simulink model "updated_target_driver_2026_withVariants_MPC"  (R2024b)
settings: Solver=FixedStepDiscrete  StartTime=0.0  StopTime=running_time  FixedStep=dt_s  RelTol=1e-3
values from neighbouring files (symbols this model uses):
  A = gamma_2*gamma_3*Thrust_desired    [force2voltage.m]
  a2_lb = -0.25    [target_driver_setup_2022_Ctrl_V_2_4.m]    (also in target_driver_setup_2022_Ctrl_V_2_4_geometric.m; target_driver_setup_mpc_12msdelay.m; target_driver_setup_mpc_andWLQP.m)
  a2_openloop = -0    (= 0)    [target_driver_setup_2022_Ctrl_V_2_4.m]    (also in target_driver_setup_2022_Ctrl_V_2_4_geometric.m; target_driver_setup_mpc_12msdelay.m; target_driver_setup_mpc_andWLQP.m)
  a2_ub = 0.25    [target_driver_setup_2022_Ctrl_V_2_4.m]    (also in target_driver_setup_2022_Ctrl_V_2_4_geometric.m; target_driver_setup_mpc_12msdelay.m; target_driver_setup_mpc_andWLQP.m)
  adaptive_flag = 0    [target_driver_setup_2022_Ctrl_V_2_4.m]    (also in target_driver_setup_2022_Ctrl_V_2_4_geometric.m; target_driver_setup_mpc_12msdelay.m = 1; target_driver_setup_mpc_andWLQP.m = 1)
  adaptive_gain = [gamma_adaptive, adaptive_roll_limit, adaptive_pitch_limit, adaptive_yaw_limit, c_2_adaptive, gamma_lateral_adaptive, adaptive_x_limit, adaptive_y_limit, adaptive_z_limit, c_1_adaptive]    [target_driver_setup_2022_Ctrl_V_2_4.m]    (also in target_driver_setup_2022_Ctrl_V_2_4_geometric.m; target_driver_setup_mpc_12msdelay.m; target_driver_setup_mpc_andWLQP.m)
  adaptive_lateral_flag = 0    [target_driver_setup_2022_Ctrl_V_2_4.m]    (also in target_driver_setup_2022_Ctrl_V_2_4_geometric.m; target_driver_setup_mpc_12msdelay.m = 1; target_driver_setup_mpc_andWLQP.m = 1)
  adaptive_pitch_init = 0    [target_driver_setup_2022_Ctrl_V_2_4.m]    (also in target_driver_setup_2022_Ctrl_V_2_4_geometric.m; target_driver_setup_mpc_12msdelay.m; target_driver_setup_mpc_andWLQP.m)
  adaptive_pitch_limit = 0.1/(scale^2)    (= 1e-07)    [target_driver_setup_2022_Ctrl_V_2_4.m]    (also in target_driver_setup_2022_Ctrl_V_2_4_geometric.m = 3e-07; target_driver_setup_mpc_12msdelay.m; target_driver_setup_mpc_andWLQP.m)
  adaptive_pitch_limit_low = -adaptive_pitch_limit    (= -1e-07)    [target_driver_setup_2022_Ctrl_V_2_4.m]    (also in target_driver_setup_2022_Ctrl_V_2_4_geometric.m = -3e-07; target_driver_setup_mpc_12msdelay.m; target_driver_setup_mpc_andWLQP.m)
  adaptive_roll_init = 0    [target_driver_setup_2022_Ctrl_V_2_4.m]    (also in target_driver_setup_2022_Ctrl_V_2_4_geometric.m; target_driver_setup_mpc_12msdelay.m; target_driver_setup_mpc_andWLQP.m)
  adaptive_roll_limit = 0.3/(scale^2)    (= 3e-07)    [target_driver_setup_2022_Ctrl_V_2_4.m]    (also in target_driver_setup_2022_Ctrl_V_2_4_geometric.m; target_driver_setup_mpc_12msdelay.m; target_driver_setup_mpc_andWLQP.m)
  adaptive_roll_limit_low = -adaptive_roll_limit    (= -3e-07)    [target_driver_setup_2022_Ctrl_V_2_4.m]    (also in target_driver_setup_2022_Ctrl_V_2_4_geometric.m; target_driver_setup_mpc_12msdelay.m; target_driver_setup_mpc_andWLQP.m)
  adaptive_x_init = 0    [target_driver_setup_2022_Ctrl_V_2_4.m]    (also in target_driver_setup_2022_Ctrl_V_2_4_geometric.m; target_driver_setup_mpc_12msdelay.m; target_driver_setup_mpc_andWLQP.m)
  adaptive_x_limit = 0.15/(scale)    (= 0.00015)    [target_driver_setup_2022_Ctrl_V_2_4.m]    (also in target_driver_setup_2022_Ctrl_V_2_4_geometric.m = 7.5e-05; target_driver_setup_mpc_12msdelay.m; target_driver_setup_mpc_andWLQP.m)
  adaptive_x_limit_low = -adaptive_x_limit    (= -0.00015)    [target_driver_setup_2022_Ctrl_V_2_4.m]    (also in target_driver_setup_2022_Ctrl_V_2_4_geometric.m = -7.5e-05; target_driver_setup_mpc_12msdelay.m; target_driver_setup_mpc_andWLQP.m)
  adaptive_y_init = 0    [target_driver_setup_2022_Ctrl_V_2_4.m]    (also in target_driver_setup_2022_Ctrl_V_2_4_geometric.m; target_driver_setup_mpc_12msdelay.m; target_driver_setup_mpc_andWLQP.m)
  adaptive_y_limit = 0.15/(scale)    (= 0.00015)    [target_driver_setup_2022_Ctrl_V_2_4.m]    (also in target_driver_setup_2022_Ctrl_V_2_4_geometric.m = 7.5e-05; target_driver_setup_mpc_12msdelay.m; target_driver_setup_mpc_andWLQP.m)
  adaptive_y_limit_low = -adaptive_y_limit    (= -0.00015)    [target_driver_setup_2022_Ctrl_V_2_4.m]    (also in target_driver_setup_2022_Ctrl_V_2_4_geometric.m = -7.5e-05; target_driver_setup_mpc_12msdelay.m; target_driver_setup_mpc_andWLQP.m)
  adaptive_yaw_init = 0    [target_driver_setup_2022_Ctrl_V_2_4.m]    (also in target_driver_setup_2022_Ctrl_V_2_4_geometric.m; target_driver_setup_mpc_12msdelay.m; target_driver_setup_mpc_andWLQP.m)
  adaptive_yaw_limit = 0.035/(scale^2)    (= 3.5e-08)    [target_driver_setup_2022_Ctrl_V_2_4.m]    (also in target_driver_setup_2022_Ctrl_V_2_4_geometric.m; target_driver_setup_mpc_12msdelay.m; target_driver_setup_mpc_andWLQP.m)
  adaptive_yaw_limit_low = -adaptive_yaw_limit    (= -3.5e-08)    [target_driver_setup_2022_Ctrl_V_2_4.m]    (also in target_driver_setup_2022_Ctrl_V_2_4_geometric.m; target_driver_setup_mpc_12msdelay.m; target_driver_setup_mpc_andWLQP.m)
  adaptive_z_init = 0/scale    (= 0)    [target_driver_setup_2022_Ctrl_V_2_4.m]    (also in target_driver_setup_2022_Ctrl_V_2_4_geometric.m; target_driver_setup_mpc_12msdelay.m; target_driver_setup_mpc_andWLQP.m)
  adaptive_z_limit = 0.20/(scale)    (= 0.0002)    [target_driver_setup_2022_Ctrl_V_2_4.m]    (also in target_driver_setup_2022_Ctrl_V_2_4_geometric.m = 0.0008; target_driver_setup_mpc_12msdelay.m = 0.0008; target_driver_setup_mpc_andWLQP.m = 0.0008)
  adaptive_z_limit_low = -adaptive_z_limit/1    (= -0.0002)    [target_driver_setup_2022_Ctrl_V_2_4.m]    (also in target_driver_setup_2022_Ctrl_V_2_4_geometric.m = -0.0008; target_driver_setup_mpc_12msdelay.m = -0.0008; target_driver_setup_mpc_andWLQP.m = -0.0008)
  att_s = 500    [target_driver_setup_2022_Ctrl_V_2_4.m]    (also in target_driver_setup_2022_Ctrl_V_2_4_geometric.m; target_driver_setup_mpc_12msdelay.m; target_driver_setup_mpc_andWLQP.m)
  b_1_d_desired = [1,0,0]    [target_driver_setup_2022_Ctrl_V_2_4.m]    (also in target_driver_setup_2022_Ctrl_V_2_4_geometric.m; target_driver_setup_mpc_12msdelay.m; target_driver_setup_mpc_andWLQP.m)
  closedloop_flag = 1    [target_driver_setup_2022_Ctrl_V_2_4.m]    (also in target_driver_setup_2022_Ctrl_V_2_4_geometric.m = 0; target_driver_setup_mpc_12msdelay.m = 0; target_driver_setup_mpc_andWLQP.m = 0)
  control_gain = [k_x,k_v, k_R, k_Omega, k_z, k_vz, k_Rx]    [target_driver_setup_2022_Ctrl_V_2_4.m]    (also in target_driver_setup_2022_Ctrl_V_2_4_geometric.m = [k_x,k_v,k_R,k_Omega_pitch,k_Omega_roll,k_z,k_vz,k_Rx]; target_driver_setup_mpc_12msdelay.m = [k_x, k_v, k_R, k_Omega, k_z, k_vz, k_Rx,                  k; target_driver_setup_mpc_andWLQP.m = [k_x, k_v, k_R, k_Omega, k_z, k_vz, k_Rx,                  k)
  delay = delay-vicon_sample_cycle/2    [target_driver_setup_2022_Ctrl_V_2_4.m]    (also in target_driver_setup_2022_Ctrl_V_2_4_geometric.m; target_driver_setup_mpc_12msdelay.m; target_driver_setup_mpc_andWLQP.m)
  drv_amp = abs((vleft_p2p-vright_p2p))/2+min(vleft_p2p,vright_p2p)    [Wing_traj_to_Voltage.m]    (also in force2voltage.m; target_driver_setup_2022_Ctrl_V_2_4.m = 300; target_driver_setup_2022_Ctrl_V_2_4_geometric.m = 133; target_driver_setup_mpc_12msdelay.m = 150)
  drv_bias = max_drv_bias    (= 300)    [target_driver_setup_2022_Ctrl_V_2_4.m]    (also in target_driver_setup_2022_Ctrl_V_2_4_geometric.m = 200; target_driver_setup_mpc_12msdelay.m = 200; target_driver_setup_mpc_andWLQP.m = 200)
  drv_pitch_left = vleft_pitch    [Wing_traj_to_Voltage.m]    (also in force2voltage.m = 0; target_driver_setup_2022_Ctrl_V_2_4.m = 0; target_driver_setup_2022_Ctrl_V_2_4_geometric.m = 0; target_driver_setup_mpc_12msdelay.m = 9.05)
  drv_pitch_right = vright_pitch    [Wing_traj_to_Voltage.m]    (also in force2voltage.m = 0; target_driver_setup_2022_Ctrl_V_2_4.m = 0; target_driver_setup_2022_Ctrl_V_2_4_geometric.m = 0; target_driver_setup_mpc_12msdelay.m = 9.05)
  drv_roll = (vleft_p2p-vright_p2p)/4    [Wing_traj_to_Voltage.m]    (also in force2voltage.m; target_driver_setup_2022_Ctrl_V_2_4.m = 0; target_driver_setup_2022_Ctrl_V_2_4_geometric.m = -0.001; target_driver_setup_mpc_12msdelay.m = -0.001)
  dt_s = 1e-3    (= 0.001)    [target_driver_setup_2022_Ctrl_V_2_4.m]    (also in target_driver_setup_2022_Ctrl_V_2_4_geometric.m = 0.0002; target_driver_setup_mpc_12msdelay.m = 0.0002; target_driver_setup_mpc_andWLQP.m = 0.0002)
  f_fin = f    (= 180)    [target_driver_setup_2022_Ctrl_V_2_4.m]    (also in target_driver_setup_2022_Ctrl_V_2_4_geometric.m = 155; target_driver_setup_mpc_12msdelay.m = 155; target_driver_setup_mpc_andWLQP.m = 155)
  f_int = f    (= 180)    [target_driver_setup_2022_Ctrl_V_2_4.m]    (also in target_driver_setup_2022_Ctrl_V_2_4_geometric.m = 155; target_driver_setup_mpc_12msdelay.m = 155; target_driver_setup_mpc_andWLQP.m = 155)
  g = 9.8    [target_driver_setup_2022_Ctrl_V_2_4.m]    (also in target_driver_setup_2022_Ctrl_V_2_4_geometric.m; target_driver_setup_mpc_12msdelay.m; target_driver_setup_mpc_andWLQP.m = 9.81; test_full_attitude_mpc.m = 9.81)
  I_moment_vec = [Ixx, Iyy, Izz]    [target_driver_setup_2022_Ctrl_V_2_4.m]    (also in target_driver_setup_2022_Ctrl_V_2_4_geometric.m; target_driver_setup_mpc_12msdelay.m; target_driver_setup_mpc_andWLQP.m)
  k_tau_vec = [k_tau_roll;k_tau_pitch]    [target_driver_setup_2022_Ctrl_V_2_4_geometric.m]    (also in target_driver_setup_mpc_12msdelay.m; target_driver_setup_mpc_andWLQP.m)
  landing_flag = 0    [target_driver_setup_2022_Ctrl_V_2_4.m]    (also in target_driver_setup_2022_Ctrl_V_2_4_geometric.m; target_driver_setup_mpc_12msdelay.m; target_driver_setup_mpc_andWLQP.m)
  landing_parameter = [start_delay+T,transition_rate, rising_time, falling_time, landing_rising_time, landing_z_decrease, landing_y_decrease, landing_x_decrease]    [target_driver_setup_2022_Ctrl_V_2_4.m]    (also in target_driver_setup_2022_Ctrl_V_2_4_geometric.m; target_driver_setup_mpc_12msdelay.m; target_driver_setup_mpc_andWLQP.m)
  low_bound = -8    [target_driver_setup_2022_Ctrl_V_2_4.m]    (also in target_driver_setup_2022_Ctrl_V_2_4_geometric.m = -5; target_driver_setup_mpc_12msdelay.m = -10; target_driver_setup_mpc_andWLQP.m = -10)
  low_bound_eR = -0.8    [target_driver_setup_2022_Ctrl_V_2_4.m]    (also in target_driver_setup_2022_Ctrl_V_2_4_geometric.m = -1.2; target_driver_setup_mpc_12msdelay.m = -1.2; target_driver_setup_mpc_andWLQP.m = -1.2)
  low_bound_vx = -0.5    [target_driver_setup_2022_Ctrl_V_2_4.m]    (also in target_driver_setup_2022_Ctrl_V_2_4_geometric.m; target_driver_setup_mpc_12msdelay.m; target_driver_setup_mpc_andWLQP.m)
  low_bound_vy = -0.5    [target_driver_setup_2022_Ctrl_V_2_4.m]    (also in target_driver_setup_2022_Ctrl_V_2_4_geometric.m; target_driver_setup_mpc_12msdelay.m; target_driver_setup_mpc_andWLQP.m)
  low_bound_vz = -0.5    [target_driver_setup_2022_Ctrl_V_2_4.m]    (also in target_driver_setup_2022_Ctrl_V_2_4_geometric.m; target_driver_setup_mpc_12msdelay.m; target_driver_setup_mpc_andWLQP.m)
  low_bound_x = -0.06    [target_driver_setup_2022_Ctrl_V_2_4.m]    (also in target_driver_setup_2022_Ctrl_V_2_4_geometric.m = -0.1; target_driver_setup_mpc_12msdelay.m = -0.6; target_driver_setup_mpc_andWLQP.m = -0.6)
  low_bound_y = -0.06    [target_driver_setup_2022_Ctrl_V_2_4.m]    (also in target_driver_setup_2022_Ctrl_V_2_4_geometric.m; target_driver_setup_mpc_12msdelay.m = -0.6; target_driver_setup_mpc_andWLQP.m = -0.6)
  low_bound_z = -0.04    [target_driver_setup_2022_Ctrl_V_2_4.m]    (also in target_driver_setup_2022_Ctrl_V_2_4_geometric.m; target_driver_setup_mpc_12msdelay.m = -0.1; target_driver_setup_mpc_andWLQP.m = -0.1)
  m = t <= t_zoom    [plot_roll_torque_cmd_vs_actual.m]    (also in plot_roll_torque_cmd_vs_actual_flightlog.m = t >= t0 & t <= t1; target_driver_setup_2022_Ctrl_V_2_4.m = 0.000124; target_driver_setup_2022_Ctrl_V_2_4_geometric.m = 8.5655e-05; target_driver_setup_mpc_12msdelay.m = 8.5655e-05)
  params_vec = [params_opt.delta_1, params_opt.delta_2, params_opt.delta_3,      params_opt.gamma_1, params_opt.gamma_2_1, params_opt.gamma_3,      params_opt.eta, params_opt.nu, params_opt.mu]'    [force2voltage_tuningSandbox.m]    (also in target_driver_setup_2022_Ctrl_V_2_4.m = [params_opt.delta_1, params_opt.delta_2, params_opt.delta_3,; target_driver_setup_2022_Ctrl_V_2_4_geometric.m = [params_opt.delta_1, params_opt.delta_2, params_opt.delta_3,; target_driver_setup_mpc_12msdelay.m = [params_opt.delta_1, params_opt.delta_2, params_opt.delta_3,; target_driver_setup_mpc_andWLQP.m = [params_opt.delta_1, params_opt.delta_2, params_opt.delta_3,)
  phase = 0    [target_driver_setup_2022_Ctrl_V_2_4.m]    (also in target_driver_setup_2022_Ctrl_V_2_4_geometric.m; target_driver_setup_mpc_12msdelay.m; target_driver_setup_mpc_andWLQP.m)
  r_desired = [default_x, default_y,z_desired]    [target_driver_setup_2022_Ctrl_V_2_4.m]    (also in target_driver_setup_2022_Ctrl_V_2_4_geometric.m; target_driver_setup_mpc_12msdelay.m; target_driver_setup_mpc_andWLQP.m)
  roll_offset_angle = 0    [target_driver_setup_2022_Ctrl_V_2_4.m]    (also in target_driver_setup_2022_Ctrl_V_2_4_geometric.m; target_driver_setup_mpc_12msdelay.m; target_driver_setup_mpc_andWLQP.m)
  running_time = start_delay+total_T    (= 9)    [target_driver_setup_2022_Ctrl_V_2_4.m]    (also in target_driver_setup_2022_Ctrl_V_2_4_geometric.m = 10; target_driver_setup_mpc_12msdelay.m = 0.5; target_driver_setup_mpc_andWLQP.m = 10)
  running_time_control = start_delay_control+total_T+0.0    (= 7.1)    [target_driver_setup_2022_Ctrl_V_2_4.m]    (also in target_driver_setup_2022_Ctrl_V_2_4_geometric.m = 10; target_driver_setup_mpc_12msdelay.m = 0.5; target_driver_setup_mpc_andWLQP.m = 10)
  sampling_f = 10000    [target_driver_setup_2022_Ctrl_V_2_4.m]    (also in target_driver_setup_2022_Ctrl_V_2_4_geometric.m = 5000; target_driver_setup_mpc_12msdelay.m = 5000; target_driver_setup_mpc_andWLQP.m = 5000)
  start_delay = 2.0    (= 2)    [target_driver_setup_2022_Ctrl_V_2_4.m]    (also in target_driver_setup_2022_Ctrl_V_2_4_geometric.m = 0; target_driver_setup_mpc_12msdelay.m = 0; target_driver_setup_mpc_andWLQP.m = 0)
  start_delay_control = start_delay + ramp_delay    (= 0.1)    [target_driver_setup_2022_Ctrl_V_2_4.m]    (also in target_driver_setup_2022_Ctrl_V_2_4_geometric.m = 0; target_driver_setup_mpc_12msdelay.m = 0; target_driver_setup_mpc_andWLQP.m = 0)
  T = 1    [target_driver_setup_2022_Ctrl_V_2_4.m]    (also in target_driver_setup_2022_Ctrl_V_2_4_geometric.m = 10; target_driver_setup_mpc_12msdelay.m = 0.5; target_driver_setup_mpc_andWLQP.m = 10; test_full_attitude_mpc.m = T0 + nu(1))
  task_flag = 0    [target_driver_setup_2022_Ctrl_V_2_4.m]    (also in target_driver_setup_2022_Ctrl_V_2_4_geometric.m; target_driver_setup_mpc_12msdelay.m; target_driver_setup_mpc_andWLQP.m)
  task_parameter = [radius_ref, frequency_ref, radius_ratio, lissajous_ratio, lissajous_delta, lissajous_amplitude_ratio,z_radius_ratio]    [target_driver_setup_2022_Ctrl_V_2_4.m]    (also in target_driver_setup_2022_Ctrl_V_2_4_geometric.m; target_driver_setup_mpc_12msdelay.m; target_driver_setup_mpc_andWLQP.m)
  upp_bound = 8    [target_driver_setup_2022_Ctrl_V_2_4.m]    (also in target_driver_setup_2022_Ctrl_V_2_4_geometric.m = 5; target_driver_setup_mpc_12msdelay.m = 10; target_driver_setup_mpc_andWLQP.m = 10)
  upp_bound_eR = 0.8    [target_driver_setup_2022_Ctrl_V_2_4.m]    (also in target_driver_setup_2022_Ctrl_V_2_4_geometric.m = 1.2; target_driver_setup_mpc_12msdelay.m = 1.2; target_driver_setup_mpc_andWLQP.m = 1.2)
  upp_bound_vx = 0.5    [target_driver_setup_2022_Ctrl_V_2_4.m]    (also in target_driver_setup_2022_Ctrl_V_2_4_geometric.m; target_driver_setup_mpc_12msdelay.m; target_driver_setup_mpc_andWLQP.m)
  upp_bound_vy = 0.5    [target_driver_setup_2022_Ctrl_V_2_4.m]    (also in target_driver_setup_2022_Ctrl_V_2_4_geometric.m; target_driver_setup_mpc_12msdelay.m; target_driver_setup_mpc_andWLQP.m)
  upp_bound_vz = 0.5    [target_driver_setup_2022_Ctrl_V_2_4.m]    (also in target_driver_setup_2022_Ctrl_V_2_4_geometric.m; target_driver_setup_mpc_12msdelay.m; target_driver_setup_mpc_andWLQP.m)
  upp_bound_x = 0.06    [target_driver_setup_2022_Ctrl_V_2_4.m]    (also in target_driver_setup_2022_Ctrl_V_2_4_geometric.m = 0.1; target_driver_setup_mpc_12msdelay.m = 0.6; target_driver_setup_mpc_andWLQP.m = 0.6)
  upp_bound_y = 0.06    [target_driver_setup_2022_Ctrl_V_2_4.m]    (also in target_driver_setup_2022_Ctrl_V_2_4_geometric.m; target_driver_setup_mpc_12msdelay.m = 0.6; target_driver_setup_mpc_andWLQP.m = 0.6)
  upp_bound_z = 0.04    [target_driver_setup_2022_Ctrl_V_2_4.m]    (also in target_driver_setup_2022_Ctrl_V_2_4_geometric.m; target_driver_setup_mpc_12msdelay.m = 0.1; target_driver_setup_mpc_andWLQP.m = 0.1)
  weights_vec = [ws; wds; wpr_xy;wpr_z; wpf; wvr_xy; wvr_z ... (first row only)    [target_driver_setup_2022_Ctrl_V_2_4_geometric.m]    (also in target_driver_setup_mpc_12msdelay.m; target_driver_setup_mpc_andWLQP.m)
undefined symbols (not defined in the file or in its folder): Com1, DiscIntNeverNeededParam, dspblkCoreblockFVToolHelper, gcbh, left_mapping, left_mapping_F_to_Phi, lp_den, lp_num, none, right_mapping, right_mapping_F_to_Phi, vlp_den, vlp_num
libraries: simulink x20, xpcseriallib x2, cstblocks x1, xpcnilib x1, xpcutilitieslib x1
(part 6 of 7)

== matlab function updated_target_driver_2026_withVariants_MPC/Trajectory_generation ==
  data: task_flag input; r_desired_total output; t input; v_desired_total output; x_d_ddot_total output; b_1_d_total output; com_desired input; b_1_d_desired input; task_parameter input; landing_parameter input; landing_flag input; b_1_d_previous input
function [r_desired_total, v_desired_total, x_d_ddot_total, b_1_d_total] = fcn(task_flag, t, com_desired, b_1_d_desired, task_parameter, landing_parameter, landing_flag, b_1_d_previous)
    % com_desired = desired center of mass 
    % b_1_d
	% 
	if task_flag == 1
		radius_ref = task_parameter(1);
		frequency_ref = task_parameter(2);
		r_desired = com_desired + radius_ref*[cos(frequency_ref*t);-sin(frequency_ref*t);0];
		v_desired = radius_ref*frequency_ref*[-sin(frequency_ref*t);-cos(frequency_ref*t);0];
		x_d_ddot  = radius_ref*frequency_ref^2*[-cos(frequency_ref*t);sin(frequency_ref*t);0];

		if radius_ref<1e-6
			b_1_d     = b_1_d_desired;
		else
			% Looking into the center
	% 		b_1_d     = (com_desired - r_desired)/norm(com_desired - r_desired);

			% Looking to the tangent

			b_1_d = v_desired/norm(v_desired);

			% Looking th camera
	% 		 b_1_d = b_1_d_desired;
		end

	elseif task_flag == 2 % Elipse
		radius_ref = task_parameter(1);
		frequency_ref = task_parameter(2);
		radius_ratio = task_parameter(3);

		r_desired = com_desired + radius_ref*[radius_ratio*cos(frequency_ref*t);-sin(frequency_ref*t);0];
		v_desired = radius_ref*frequency_ref*[-radius_ratio*sin(frequency_ref*t);-cos(frequency_ref*t);0];
		x_d_ddot  = radius_ref*frequency_ref^2*[-radius_ratio*cos(frequency_ref*t);-(-sin(frequency_ref*t));0];

		if radius_ref<1e-6
			b_1_d     = b_1_d_desired;
		else
			% Looking into the center
	% 		b_1_d     = (com_desired - r_desired)/norm(com_desired - r_desired);

			% Looking to the tangent

			b_1_d = v_desired/norm(v_desired);
		end
	elseif task_flag==3 % Vertical up and down with the landing
		radius_ref = task_parameter(1);
		frequency_ref = task_parameter(2);
		landing_time = landing_parameter(1);

		r_desired = com_desired + radius_ref*[0;0;sin(frequency_ref*(t-landing_time)-pi/2)];
		v_desired = radius_ref*frequency_ref*[0;0;cos(frequency_ref*(t-landing_time)-pi/2)];
		x_d_ddot  = radius_ref*frequency_ref^2*[0;0;-sin(frequency_ref*(t-landing_time)-pi/2)];

		if radius_ref<1e-6
			b_1_d     = b_1_d_desired;
		else
			% Looking into the center
	% 		b_1_d     = (com_desired - r_desired)/norm(com_desired - r_desired);

			% Looking to the tangent

	% 		b_1_d = v_desired/norm(v_desired);
			% Looking th camera
			 b_1_d = b_1_d_desired;
		end
	elseif task_flag==4 % circle in y-z landing
		radius_ref = task_parameter(1);
		frequency_ref = task_parameter(2);
		landing_time = landing_parameter(1);

		r_desired = com_desired + radius_ref*[0;cos(frequency_ref*(t-landing_time)-pi/2);sin(frequency_ref*(t-landing_time)-pi/2)];
		v_desired = radius_ref*frequency_ref*[0;-sin(frequency_ref*(t-landing_time)-pi/2);cos(frequency_ref*(t-landing_time)-pi/2)];
		x_d_ddot  = radius_ref*frequency_ref^2*[0;-cos(frequency_ref*(t-landing_time)-pi/2);-sin(frequency_ref*(t-landing_time)-pi/2)];

		if radius_ref<1e-6
			b_1_d     = b_1_d_desired;
		else
			% Looking into the center
	% 		b_1_d     = (com_desired - r_desired)/norm(com_desired - r_desired);

			% Looking to the tangent

	% 		b_1_d = v_desired/norm(v_desired);
			% Looking th camera
			 b_1_d = b_1_d_desired;
		end	
	elseif task_flag==5 % Lissajous curve in y-z landing
		radius_ref = task_parameter(1);
		frequency_ref = task_parameter(2);
		landing_time = landing_parameter(1);
		lissajous_ratio = task_parameter(4);
		lissajous_delta = task_parameter(5);
		lissajous_amplitude_ratio = task_parameter(6);

		r_desired = com_desired + radius_ref*[0;sin(frequency_ref*lissajous_ratio*(t-landing_time)+lissajous_delta)											;lissajous_amplitude_ratio*sin(frequency_ref*(t-landing_time))];
		v_desired = radius_ref*frequency_ref*[0;lissajous_ratio*cos(frequency_ref*lissajous_ratio*(t-landing_time)+lissajous_delta)			;lissajous_amplitude_ratio*cos(frequency_ref*(t-landing_time))];
		x_d_ddot  = radius_ref*frequency_ref^2*[0;-lissajous_ratio^2*sin(frequency_ref*lissajous_ratio*(t-landing_time)+lissajous_delta)	;-lissajous_amplitude_ratio*sin(frequency_ref*(t-landing_time))];

		if radius_ref<1e-6
			b_1_d     = b_1_d_desired;
		else

			% Looking th camera
			 b_1_d = b_1_d_desired;
		end

	elseif task_flag==6 % Elipse
		radius_ref = task_parameter(1);
		frequency_ref = task_parameter(2);
		radius_ratio = task_parameter(3);
		z_radius_ratio = task_parameter(7);

		r_desired = com_desired + radius_ref*[radius_ratio*cos(frequency_ref*t);-sin(frequency_ref*t);-z_radius_ratio*sin(frequency_ref*t)];
		v_desired = radius_ref*frequency_ref*[-radius_ratio*sin(frequency_ref*t);-cos(frequency_ref*t);-z_radius_ratio*cos(frequency_ref*t)];
		x_d_ddot  = radius_ref*frequency_ref^2*[-radius_ratio*cos(frequency_ref*t);-(-sin(frequency_ref*t));-z_radius_ratio*(-sin(frequency_ref*t))];

		if radius_ref<1e-6
			b_1_d     = b_1_d_desired;
		else
			% Looking into the center
	% 		b_1_d     = (com_desired - r_desired)/norm(com_desired - r_desired);

			% Looking to the tangent

			b_1_d = v_desired/norm(v_desired);
		end	

	elseif task_flag==7 % Elipse
		radius_ref = task_parameter(1);
		heading_vector = [0;-1;0];

		r_desired = com_desired + radius_ref*heading_vector;
		v_desired = [0;0;0];
		x_d_ddot  = [0;0;0];

		if radius_ref<1e-6
			b_1_d     = b_1_d_desired;
		else
			% Looking into the center
	% 		b_1_d     = (com_desired - r_desired)/norm(com_desired - r_desired);

			% Looking to the tangent

	% 		b_1_d = v_desired/norm(v_desired);
			% Looking at the camera
			b_1_d     = b_1_d_desired;

		end		
	elseif task_flag==8
		landing_y_decrease = landing_parameter(7);
		landing_x_decrease = landing_parameter(8);

		r_desired = com_desired+[landing_x_decrease;landing_y_decrease;0];
		v_desired = [0;0;0];
		x_d_ddot  = [0;0;0];
		b_1_d     = b_1_d_desired;

	else
		r_desired = com_desired;
		v_desired = [0;0;0];
		x_d_ddot  = [0;0;0];
		b_1_d     = b_1_d_desired;
	end

	if landing_flag==1

		trans_rate=landing_parameter(2);
		rising_time =landing_parameter(3);
		falling_time =landing_parameter(4);
		landing_rising_time = landing_parameter(5);
		landing_z_decrease = landing_parameter(6);
		landing_y_decrease = landing_parameter(7);
		landing_x_decrease = landing_parameter(8);

	% Referenece trajectory band-pass

		if task_flag==8
			rising_func = (1+tanh(trans_rate*(t-rising_time)))/2;
			fallilng_func = 0;

		else
			rising_func = (1+tanh(trans_rate*(t-rising_time)))/2-1/2;
			fallilng_func = (1-tanh(trans_rate*(t-falling_time)))/2-1/2;

		end

		landing_rising_func = (1+tanh(trans_rate*(t-landing_rising_time)))/2;

		bandpass_func = rising_func+fallilng_func;
		neg_bandpass_func = -bandpass_func+1;

		der_bandpass_func = trans_rate*(1 -(tanh(trans_rate*(t-rising_time))).^2)/2 -trans_rate*(1-(tanh(trans_rate*(t-falling_time))).^2)/2;
		dder_bandpass_func = -2*trans_rate^2*(tanh(trans_rate*(t-rising_time))).*(1 -(tanh(trans_rate*(t-rising_time))).^2)/2 +2*trans_rate^2*(tanh(trans_rate*(t-falling_time))).*(1-(tanh(trans_rate*(t-falling_time))).^2)/2;

		der_landing_func = trans_rate*(1 -(tanh(trans_rate*(t-landing_rising_time))).^2)/2;
		dder_landing_func = -2*trans_rate^2*(tanh(trans_rate*(t-landing_rising_time))).*(1 -(tanh(trans_rate*(t-landing_rising_time))).^2)/2;

		landing_desired = com_desired+[landing_x_decrease;landing_y_decrease;landing_z_decrease];
	% 	landing_desired = com_desired+[0;0;landing_z_decrease];

		if task_flag==8 % Landing only z direction at r_desired point
			r_desired_total = com_desired + bandpass_func.*(r_desired-com_desired)+landing_rising_func.*(landing_desired-r_desired);
		else
			r_desired_total = com_desired + bandpass_func.*(r_desired-com_desired)+landing_rising_func.*(landing_desired-com_desired);	
		end

		v_desired_total = der_bandpass_func.*(r_desired-com_desired) + bandpass_func.*v_desired + der_landing_func.*(landing_desired-com_desired);
		x_d_ddot_total = dder_bandpass_func.*(r_desired-com_desired) + 2*der_bandpass_func.*v_desired+ bandpass_func.*x_d_ddot+ dder_landing_func.*(landing_desired-com_desired);

	% Heading trajectory band-pass
		trans_heading_rate = trans_rate*1/1;
		rising_heading_func = (1+tanh(trans_heading_rate*(t-(rising_time+1))))/2-1/2;
		fallilng_heading_func = (1-tanh(trans_heading_rate*(t-falling_time+1)))/2-1/2;
	% rising_heading_func = (1+tanh(trans_heading_rate*(t-(rising_time))))/2-1/2;
	% 	fallilng_heading_func = (1-tanh(trans_heading_rate*(t-falling_time)))/2-1/2;


		bandpass_heading_func = rising_heading_func+fallilng_heading_func;
		neg_bandpass_heading_func = -bandpass_heading_func+1;
		landing_rising_heading_func = (1+tanh(trans_heading_rate*(t-landing_rising_time)))/2;
	% 
	% 	if norm(v_desired_total)<1e-6
	% 		b_1_d     = b_1_d_desired;
	% 	else
	% 		b_1_d = v_desired_total/norm(v_desired_total);
	% 	end
	% 	
	% 	b_1_d_total = b_1_d_desired.*neg_bandpass_heading_func + b_1_d.*bandpass_heading_func;
	% 	
	% 	b_1_d_total = b_1_d_total/norm(b_1_d_total);
	% 	
	% 		% Convex combination of the heading vector
	% 	% Linear convex comb
	% 	b_1_d_total = b_1_d_desired.*neg_bandpass_func + b_1_d.*bandpass_func;


	% Slerp for smooth heading transition
	% STEP 1 : Hovering to Desired trajectory to Hovering

		if t<rising_time && bandpass_heading_func<1e-5%1e-6
			b_1_d_current = b_1_d_desired;
		else
			b_1_d_current = b_1_d_previous;
		end


		cos_Omega_slerp = b_1_d.'*b_1_d_current;
		Omega_slerp = acos(cos_Omega_slerp);

		if Omega_slerp<1e-8
			b_1_d_total = b_1_d_current.*neg_bandpass_heading_func + b_1_d.*bandpass_heading_func;
		else
			b_1_d_total = sin(neg_bandpass_heading_func*Omega_slerp)/sin(Omega_slerp)*b_1_d_current + sin(bandpass_heading_func*Omega_slerp)/sin(Omega_slerp)*b_1_d;
		end

	% STEP 2 : Hovering to Desired Heading for landing

		b_1_d_total = sin(1-landing_rising_heading_func)*b_1_d_total + sin(landing_rising_heading_func)*b_1_d_desired;

		b_1_d_total = b_1_d_total/norm(b_1_d_total);

	else
		r_desired_total = r_desired;
		v_desired_total = v_desired;
		x_d_ddot_total = x_d_ddot;
		b_1_d_total = b_1_d;

	end
end

== matlab function updated_target_driver_2026_withVariants_MPC/Force_to_Voltage1/Trajectory to Voltage Input  ==
  data: Phi_left_p2p_command input; drv_amp output; Phi_right_p2p_command input; Phi_pitch_command input; drv_roll output; drv_pitch_left output; left_mapping input; right_mapping input; drv_pitch_right output
function [drv_amp, drv_roll, drv_pitch_left, drv_pitch_right] = fcn(Phi_left_p2p_command,Phi_right_p2p_command,Phi_pitch_command,left_mapping,right_mapping)

% Mapping for Voltage peak to peak from desired Stroke peak to peak
p1_left = left_mapping(1); % V_left_p2p = p1_left*Phi_p2p + p2_left
p2_left = left_mapping(2);
p1_right = right_mapping(1); % V_right_p2p = p1_right*Phi_p2p + p2_right
p2_right = right_mapping(2);

% Mapping for Voltage offset to peak from desired Stroke peak to peak
p1_pitch_left = left_mapping(3); % vleft_pitch = p1_pitch_left*Phi_pitch_command + p2_pitch_left
p2_pitch_left = left_mapping(4);
p1_pitch_right = right_mapping(3); % vright_pitch = p1_pitch_right*Phi_pitch_command + p2_pitch_right
p2_pitch_right = right_mapping(4);

vleft_p2p = p1_left*Phi_left_p2p_command + p2_left;
vright_p2p = p1_right*Phi_right_p2p_command + p2_right;
vleft_pitch = p1_pitch_left*Phi_pitch_command + p2_pitch_left;
vright_pitch = p1_pitch_right*Phi_pitch_command + p2_pitch_right;



drv_amp = abs((vleft_p2p-vright_p2p))/2+min(vleft_p2p,vright_p2p); % p2p
drv_roll = (vleft_p2p-vright_p2p)/4; % Amplitude
drv_pitch_left = vleft_pitch;
drv_pitch_right = vright_pitch;

== matlab function updated_target_driver_2026_withVariants_MPC/Observer for averaged system1/Attitude Observer/Geometric Averaging Rotation Matix/Averaged quaternion ==
  data: R input; quat output
function quat = fcn(R)
Rot = zeros(3,3);
Rot = [R(1), R(2), R(3); R(4), R(5), R(6); R(7), R(8), R(9); ];
quat = rotm2quat(Rot)';

== matlab function updated_target_driver_2026_withVariants_MPC/Observer for averaged system1/Attitude Observer/Geometric Averaging Rotation Matix/Geometric Averaging Rotation M/Geometric Average  ==
  data: R_prev input; R_prev2 input; R_prev3 input; R_prev4 input; R_prev5 input; R_prev6 input; Rout output; R_cur input; update input; Rout_prev input
function Rout = fcn(R_prev,R_prev2,R_prev3,R_prev4,R_prev5,R_prev6,R_cur,update,Rout_prev)
%#codegen
% Average recent rotation matrices safely near small angles.
%
% Inputs are 9-vectors using row-major packing:
% R_vec = [R(1,1); R(1,2); R(1,3);
%          R(2,1); R(2,2); R(2,3);
%          R(3,1); R(3,2); R(3,3)]
%
% Output uses the same row-major packing.

Rout = zeros(9,1);

R_cur      = reshape(R_cur,9,1);
R_prev     = reshape(R_prev,9,1);
R_prev2    = reshape(R_prev2,9,1);
R_prev3    = reshape(R_prev3,9,1);
R_prev4    = reshape(R_prev4,9,1); %#ok<NASGU>
R_prev5    = reshape(R_prev5,9,1); %#ok<NASGU>
R_prev6    = reshape(R_prev6,9,1); %#ok<NASGU>
Rout_prev  = reshape(Rout_prev,9,1);

% Reconstruct row-major 9-vector into 3x3 matrix.
Rot_cur   = vec_to_rotm(R_cur);
Rot_prev  = vec_to_rotm(R_prev);
Rot_prev2 = vec_to_rotm(R_prev2);
Rot_prev3 = vec_to_rotm(R_prev3);

if update > 0
    Rout = Rout_prev;
else
    % 1-cycle / 4-sample average.
    %
    % IMPORTANT:
    % Do not do sign correction like w = -w here.
    % That is valid for quaternions, but not for rotation vectors.
    w_R0 = log_so3(Rot_cur);
    w_R1 = log_so3(Rot_prev);
    w_R2 = log_so3(Rot_prev2);
    w_R3 = log_so3(Rot_prev3);

    w_mean = (w_R0 + w_R1 + w_R2 + w_R3) / 4.0;

    mean_R = exp_so3(w_mean);

    % Optional but useful: project back to SO(3) to remove tiny numerical drift.
    mean_R = project_to_so3(mean_R);

    Rout = rotm_to_vec(mean_R);
end

end


function R = vec_to_rotm(R_vec)
% Convert row-major 9-vector to 3x3 matrix.

R = [R_vec(1), R_vec(2), R_vec(3);
     R_vec(4), R_vec(5), R_vec(6);
     R_vec(7), R_vec(8), R_vec(9)];
end


function R_vec = rotm_to_vec(R)
% Convert 3x3 matrix to row-major 9-vector.

R_vec = [R(1,1);
         R(1,2);
         R(1,3);
         R(2,1);
         R(2,2);
         R(2,3);
         R(3,1);
         R(3,2);
         R(3,3)];
end


function w = log_so3(R)
% Small-angle-safe logarithm map from SO(3) to rotation vector.
%
% For small theta, avoid theta/(sin(theta)) numerical issues.

c = (trace(R) - 1.0) / 2.0;

% Clamp for numerical safety.
if c > 1.0
    c = 1.0;
elseif c < -1.0
    c = -1.0;
end

theta = acos(c);

vee_part = [R(3,2) - R(2,3);
            R(1,3) - R(3,1);
            R(2,1) - R(1,2)];

if theta < 1.0e-6
    % Since R - R' ~= 2*w_hat for small rotations.
    w = 0.5 * vee_part;
else
    s = sin(theta);

    if abs(s) < 1.0e-9
        % Near pi is not expected in hover, but this avoids division blow-up.
        % Fall back to small-angle style approximation rather than producing NaN.
        w = 0.5 * vee_part;
    else
        w = theta / (2.0 * s) * vee_part;
    end
end

end


function R = exp_so3(w)
% Small-angle-safe exponential map from rotation vector to SO(3).

theta = norm(w);

W = [0.0,   -w(3),  w(2);
     w(3),   0.0,  -w(1);
    -w(2),   w(1),  0.0];

if theta < 1.0e-6
    % Rodrigues small-angle expansion.
    R = eye(3) + W + 0.5 * (W * W);
else
    R = eye(3) ...
        + (sin(theta) / theta) * W ...
        + ((1.0 - cos(theta)) / (theta * theta)) * (W * W);
end

end


function R_out = project_to_so3(R_in)
% Project a near-rotation matrix back to SO(3).
% This prevents slow drift from numerical errors.

[U,~,V] = svd(R_in);
R_out = U * V';

if det(R_out) < 0
    U(:,3) = -U(:,3);
    R_out = U * V';
end

end

== matlab function updated_target_driver_2026_withVariants_MPC/Observer for averaged system1/Attitude Observer/Geometric Averaging Rotation Matix/Raw quaternion ==
  data: R input; quat output
function quat = fcn(R)
Rot = zeros(3,3);
Rot = [R(1), R(2), R(3); R(4), R(5), R(6); R(7), R(8), R(9); ];
quat = rotm2quat(Rot)';

== matlab function updated_target_driver_2026_withVariants_MPC/Observer for averaged system1/Attitude Observer/Geometric derivative in SO(3)/First order geometric derivative in SO(3)  ==
  data: R_prev input; omega output size=[3 1]; R_cur input; omega_prev input; update input; count input; sampling_f input
function omega  = fcn(R_prev, R_cur, omega_prev, update, count,sampling_f)

Rot_cur = [R_cur(1), R_cur(2), R_cur(3); R_cur(4), R_cur(5), R_cur(6); R_cur(7), R_cur(8), R_cur(9)];
Rot_prev = [R_prev(1), R_prev(2), R_prev(3); R_prev(4), R_prev(5), R_prev(6); R_prev(7), R_prev(8), R_prev(9)];

R_diff = Rot_prev'*Rot_cur;

tr_R_diff = trace(R_diff);
omega = zeros(3,1);
if update>0
   omega=omega_prev; 
else
    
% isreal(tr_R_diff)
if abs((tr_R_diff-1)/2)<=1
    theta = acos((tr_R_diff-1)/2);
else
    theta=acos((tr_R_diff-1)/2/abs((tr_R_diff-1)/2));
end

% To avoid NaN for omega
if theta<1e-10
	omega = omega_prev;
else
	w = 1/(2*sin(theta))*[R_diff(3,2)-R_diff(2,3); R_diff(1,3) - R_diff(3,1); R_diff(2,1)-R_diff(1,2)];

	omega = w*theta*sampling_f/(count+1);
end   

end
% 
% if theta==0 %update~=0 
%     y = y_prev;
% else
%      w = 1/(2*sin(theta))*[R_diff(3,2)-R_diff(2,3); R_diff(1,3) - R_diff(3,1); R_diff(2,1)-R_diff(1,2)];
%      y = w*theta*10000/20;
% end

== matlab function updated_target_driver_2026_withVariants_MPC/Observer for averaged system1/Euler derivative & filtered angular velocity /Angular velocity ==
  data: R input; Rdot input; w output; Frob_error output
function [w,Frob_error] = fcn(R,Rdot)
%#codegen
Rot = [R(1), R(2), R(3); R(4), R(5), R(6); R(7), R(8), R(9); ];
dRot = [Rdot(1), Rdot(2), Rdot(3); Rdot(4), Rdot(5), Rdot(6); Rdot(7), Rdot(8), Rdot(9); ];

A = Rot'*dRot;
w_hat = 1/2*(A-A');
w=zeros(3,1);
w(1) = w_hat(3,2);
w(2) = w_hat(1,3);
w(3) = w_hat(2,1);
% wz = w(3);
Frob_error=trace((A+A')*(A+A'));

== matlab function updated_target_driver_2026_withVariants_MPC/Observer for averaged system1/Position Observer/Averaging position & velocity  ==
  data: r_prev input; r_prev2 input; r_prev3 input; r_cur input; update input; count input; rout_prev input; rout output; vout_prev input; vout output; sampling_f input
function [rout, vout] = fcn(r_prev,r_prev2,r_prev3,r_cur,update, count,rout_prev,vout_prev,sampling_f)
%#codegen

rout = zeros(3,1);
vout = zeros(3,1);
if update>0
   rout=rout_prev; 
   vout=vout_prev;
else

    % 1 cycle average
    n= 4;
    
    rout = (r_prev+r_prev2+r_prev3+r_cur)/n;
    vout = (rout-rout_prev)*sampling_f/(count+1);
    
  
end

end

== matlab function updated_target_driver_2026_withVariants_MPC/Open_Closed_loop_selection/MATLAB Function ==
  data: time input; freq output; f_int parameter; f_fin parameter; T parameter
function freq = fcn(time, f_int, f_fin, T)
%#codegen

freq = f_int;
buffer_t = 0.0; %3.0
rel_time = time-buffer_t;
if rel_time > 0
    freq = f_int + (f_fin-f_int) * (rel_time/T);
end

if freq > f_fin
    freq = f_fin;
end

== matlab function updated_target_driver_2026_withVariants_MPC/Vicon Post Processing1/Vicon Validity check/MATLAB Function3 ==
  data: R_prev input; y output; R_cur input
function y = fcn(R_prev,R_cur)
Rot_cur = [R_cur(1), R_cur(2), R_cur(3); R_cur(4), R_cur(5), R_cur(6); R_cur(7), R_cur(8), R_cur(9)];
Rot_prev = [R_prev(1), R_prev(2), R_prev(3); R_prev(4), R_prev(5), R_prev(6); R_prev(7), R_prev(8), R_prev(9)];

A=Rot_cur'*Rot_prev;
epsilonn = 1e-18;

if trace((A-eye(3))'*(A-eye(3)))<epsilonn
   y=0; 
else
    y=1;
end

== matlab function updated_target_driver_2026_withVariants_MPC/Vicon Post Processing1/Vicon correction ==
  data: R_cur input; Rot_corrected_vec output; roll_offset_angle input
function Rot_corrected_vec = fcn(R_cur,roll_offset_angle)

Rot_cur = [R_cur(1), R_cur(2), R_cur(3); R_cur(4), R_cur(5), R_cur(6); R_cur(7), R_cur(8), R_cur(9)];
Rot_correction = [1, 0, 0; ...
									0, cos(roll_offset_angle), -sin(roll_offset_angle);...
									0, sin(roll_offset_angle), cos(roll_offset_angle)];
Rot_corrected = Rot_correction*Rot_cur;

Rot_corrected_vec = [Rot_corrected(1,1); Rot_corrected(1,2); Rot_corrected(1,3); Rot_corrected(2,1); Rot_corrected(2,2); Rot_corrected(2,3); Rot_corrected(3,1); Rot_corrected(3,2); Rot_corrected(3,3)];

end

== matlab function updated_target_driver_2026_withVariants_MPC/Vicon correction1 ==
  data: x_cur input; x_corrected_vec output; roll_offset_angle input
function x_corrected_vec = fcn(x_cur,roll_offset_angle)

x_cur_vec = [x_cur(1); x_cur(2); x_cur(3)];
Rot_correction = [1, 0, 0; ...
									0, cos(roll_offset_angle), -sin(roll_offset_angle);...
									0, sin(roll_offset_angle), cos(roll_offset_angle)];
x_corrected_vec = Rot_correction*x_cur_vec;

end

== matlab function updated_target_driver_2026_withVariants_MPC/Force to voltage/Control Mode/Desired_Force_to_Voltage ==
  data: Thrust_desired input; drv_amp output; Roll_torque_desired input; Pitch_torque_desired input; Yaw_torque_desired input; drv_roll output; drv_pitch_left output; drv_pitch_right output; a2_coeff output; params_vec input
function [drv_amp, drv_roll, drv_pitch_left, drv_pitch_right, a2_coeff] =    fcn(Thrust_desired, Roll_torque_desired, Pitch_torque_desired, Yaw_torque_desired, params_vec)

% 
% Thrust_desired = 0.7e-3;% N
% Roll_torque_desired = 20e-6; %mN mm 
% Pitch_torque_desired = 0;% N  
% Yaw_torque_desired = 0;  
[drv_amp, drv_roll, drv_pitch_left, drv_pitch_right, a2_coeff] = force2voltage( ...
    Thrust_desired, Roll_torque_desired, Pitch_torque_desired, ...
    Yaw_torque_desired, params_vec);
% % global params_opt
% 
% delta_1 = params_vec(1);
% delta_2 = params_vec(2);
% delta_3 = params_vec(3);
% gamma_1 = params_vec(4);
% gamma_2 = params_vec(5);
% gamma_3 = params_vec(6);
% eta = params_vec(7);
% nu = params_vec(8);
% mu = params_vec(9);
% 
% 
% % Initializing for averaging filter at the end to prevent InF
% if Thrust_desired==0    
%     u4 = 0;
% else
%     u4 = Pitch_torque_desired/(Thrust_desired*delta_3*gamma_2)-nu;
% end
% 
% 
% % u3 calculation when tau approaches to zero
% if abs(Yaw_torque_desired)<1e-12
% 
%    u3 = -mu;
% else
%     % Bounds for the mapping to produce real solution
%     lb =(Thrust_desired/2)*(gamma_2*gamma_3*delta_2*mu/delta_1-sqrt((gamma_2*gamma_3*delta_2*Thrust_desired*mu/delta_1)^2+gamma_2*gamma_3));
%     ub =(Thrust_desired/2)*(gamma_2*gamma_3*delta_2*mu/delta_1+sqrt((gamma_2*gamma_3*delta_2*Thrust_desired*mu/delta_1)^2+gamma_2*gamma_3));
% 
%     if Yaw_torque_desired>=ub
%        Yaw_torque_desired = ub;
%     elseif Yaw_torque_desired<=lb
%        Yaw_torque_desired = lb; 
%     end
% 
%     % u3 calculation when tau approaches zero
%     if abs(Yaw_torque_desired) < 1e-12
%         u3 = -mu;
%     else
%         A = gamma_2*gamma_3*Thrust_desired;
%         B = gamma_2*gamma_3*delta_2*Thrust_desired*mu/delta_1;
% 
%         disc = A^2 - 4*Yaw_torque_desired*(Yaw_torque_desired - B);
% 
%     % Numerical / feasibility guard
%     if disc < 0
%         disc = 0;
%     end
% 
%     u3 = delta_1*(A - sqrt(disc))/(2*delta_2*Yaw_torque_desired);
%     end
% end
% 
% D = delta_1^2+delta_2^2*u3^2;
% % gamma_2*Thrust_desired+Roll_torque_desired 
% u1 = (gamma_2*Thrust_desired+Roll_torque_desired)/(2*gamma_1*gamma_2*D*eta);
% u2 = (gamma_2*Thrust_desired-Roll_torque_desired)/(2*gamma_1*gamma_2*D);
% 
% u1 = max(u1, 0); 
% u2 = max(u2, 0); % Guard against negative voltage
% vleft_p2p = sqrt(u1)*2; 
% vright_p2p = sqrt(u2)*2;
% vleft_pitch = u4;
% vright_pitch = u4;
% 
% 
% drv_amp = abs((vleft_p2p-vright_p2p))/2+min(vleft_p2p,vright_p2p); % p2p
% drv_roll = (vleft_p2p-vright_p2p)/4; % Amplitude
% drv_pitch_left = vleft_pitch;
% drv_pitch_right = vright_pitch;
% a2_coeff = u3;
% 
end

== matlab function updated_target_driver_2026_withVariants_MPC/Desired body z ==
  data: x_d_ddot input; s_des output; g input
function s_des = fcn(x_d_ddot, g)
%#codegen
% Desired body-z vector for the monolithic upright MPC: the direction
% of the required specific force, g*e3 plus the trajectory feed-forward
% acceleration. Pure feed-forward -- no position feedback, no heading.
f = [0;0;g] + reshape(x_d_ddot,3,1);
n = norm(f);
if n < 1.0e-9
    s_des = [0;0;1];
else
    s_des = f/n;
end
end
